simulink model "five_bar_model_v_1"  (R2018a)
settings: Solver=ode45  StartTime=0.0  StopTime=tmax  FixedStep=0.0001  MaxStep=1e-4  RelTol=1e-3
values from neighbouring files (symbols this model uses):
  dt = 10e-3    (= 0.01)    [model_parameters_v_1.m]    (also in test_dynamics.m = 0.2; test_kinematics.m = 0.1)
  g = -9.80665    [idyn5.m]    (also in test_dynamics.m; test_model.m = 9.80665)
  Kd = (3*aj*wj-Fv) * eye(2)    [model_parameters_v_1.m]
  Kdi = [2 * zita *  wpos1; 2  * zita * wpos2]    [model_parameters_v_1.m]
  Ki = aj*wj^3 * eye(2)    [model_parameters_v_1.m]
  Kp = 3*aj*wj^2 * eye(2)    [model_parameters_v_1.m]
  Kpi = [ wpos1^2;  wpos2^2]    [model_parameters_v_1.m]
  p = [NaN; NaN]    [fkine5.m]    (also in test_model.m = zeros(n,2))
  q = [NaN; NaN; NaN; NaN; NaN]    [fkine5.m]    (also in ikine5.m = [q11;q12;q13;q21;q22])
  q0 = q(:,1)    [model_parameters_v_1.m]    (also in test_dynamics.m = q0(:,4); test_kinematics.m = q0(:,4))
  qd = [qda(1);qdu(1);qdu(2);qda(2);qdu(3)]    [ifirstkine5.m]
  qdd = [qdda(1);qddu(1);qddu(2);qdda(2);qddu(3)]    [isecondkine5.m]
  t0r = J * qda    [ffirstkine5.m]    (also in test_dynamics.m = [0;0]; test_kinematics.m = [1;1]; test_model.m = p)
  t0rd = (J * qdda+ at)    [fsecondkine5.m]    (also in test_dynamics.m = [0;0]; test_kinematics.m = [-1;1]; test_model.m = p)
undefined symbols (not defined in the file or in its folder): Kii, tmax, X, Y, Z
libraries: sm_lib x24, simulink x12, nesl_utility x9, powerlib_meascontrol x2
(part 2 of 2)

== matlab function five_bar_model_v_1/five-bar-robot1/direct dynamic ==
  data: T input; qdda output; q input; qd input; J input; Jt input; Jta input; Jtd input; Psit input; atp input; ad input; Tl input
function qdda  = ddyn5(T,q,qd,J,Jt,Jta,Jtd,Psit,atp,ad, Tl)
    l = 0.205;
    d1 = [-0.125, l, l];
    d2 = [0.125, l, l];
    q1 = q(1:3);
    q2 = q(4:5);
    qd1 = qd(1:3);
    qd2 = qd(4:5);
    % Numerical Solution Dynamics
    % Gravity 
%     g = -9.80665;
    g = 0;
    
   % Dynamics parameters
    m11 = 0.126; %kg
    mx11 = m11 * 0.1025;
    my11 =  0; %m11 * 1.44e-2;
    zz11 = 0.001774; %kg-m^2;
    
    m12 = 0.126; %kg
    mx12 = m12 * 0.1025;
    my12 =  0; %m11 * 1.44e-2;
    zz12 = 0.001774; %kg-m^2;
    
    m21 = 0.126; %kg
    mx21 = m21 * 0.1025;
    my21 =  0; %m11 * 1.44e-2;
    zz21 = 0.001774; %kg-m^2;
    
    m22 = 0.126; %kg
    mx22 = m22 * 0.1025;
    my22 =  0; %m11 * 1.44e-2;
    zz22 = 0.001774; %kg-m^2;
    
    Ia11 = 4.8e-5; % kg-m2
    zz11r = zz11 + Ia11 + d1(2)^2 * m12;
    
    Ia21 = 4.8e-5; % kg-m2
    zz21r = zz21 + Ia21 + d2(2)^2 * m22;
   
    %Fricciones fv = viscosa fs= seca
    fv1 = [1.5e-1 0 0];
    fs1 = [1.5e-1 0 0];
    fv2 = [0 0];
    fs2 = [0 0];
    % End effector mass
    m4 = 0.272;
    
    % Direct dynamics model
    M11 = zz11r + zz12 + 2 * d1(2) * mx12 * cos(q1(2)) - ...
          2 * d1(2) * my12 * sin(q1(2));

    M12 = zz12 + d1(2) * mx12 * cos(q1(2)) - ...
          d1(2) * my12 * sin(q1(2));
    M21 = M12;

    M44 = zz21r + zz22 + 2 * d2(2) * mx22 * cos(q2(2)) - ...
          2 * d2(2) * my22 * sin(q2(2));

    M45 = zz22 + d2(2) * mx22 * cos(q2(2)) - ...
          d2(2) * my22 * sin(q2(2));
    M54 = M45;

    Mt = [M11 M12  0 0     0;
          M21 zz12 0 0     0;
          0   0    0 0     0;
          0   0    0 M44 M45;
          0   0    0 M54 zz22];

    c1 = -d1(2) * mx12 * qd1(2) * (2 * qd1(1) + qd1(2)) * sin(q1(2)) ...
         -d1(2) * my12 * qd1(2) * (2 * qd1(1) + qd1(2)) * cos(q1(2)) ...
         +fs1(1) * sign(qd1(1)) + fv1(1) * qd1(1) ...
         +(my12*sin(q1(1) + q1(2)) - mx12*cos(q1(1) + q1(2)) ...
         - mx11*cos(q1(1)) + my11*sin(q1(1)) - d1(2)*m12*cos(q1(1)))*g;

    c2 = d1(2) * mx12 * qd1(1)^2 * sin(q1(2)) ...
         +d1(2) * my12 * qd1(1)^2 * cos(q1(2)) ...
         +fs1(2) * sign(qd1(2)) + fv1(2) * qd1(2) ...
         +(my12*sin(q1(1) + q1(2)) - mx12*cos(q1(1) + q1(2)))*g;

    c3 = fs1(3)*sign(qd1(3)) + fv1(3)*qd1(3);

    c4 = -d2(2) * mx22 * qd2(2) * (2 * qd2(1) + qd2(2)) * sin(q2(2)) ...
         -d2(2) * my22 * qd2(2) * (2 * qd2(1) + qd2(2)) * cos(q2(2)) ...
         +fs2(1) * sign( qd2(1) ) + fv2(1) * qd2(1) ...
         +(my22*sin(q2(1) + q2(2)) - mx22*cos(q2(1) + q2(2)) ...
         -mx21*cos(q2(1)) + my21*sin(q2(1)) - d2(2)*m22*cos(q2(1)))*g;

    c5 = d2(2) * mx22 * qd2(1)^2 * sin(q2(2)) ...
         +d2(2) * my22 * qd2(1)^2 * cos(q2(2)) ...
         +fs2(2) * sign(qd2(2)) + fv2(2) * qd2(2) ...
         +(my22*sin(q2(1) + q2(2)) - mx22*cos(q2(1) + q2(2)))*g;

    ct = [c1; c2; c3; c4; c5];

    Et = [1 0 0 0 0;
          0 0 1 0 0;
          0 0 0 1 0;
          0 1 0 0 0;
          0 0 0 0 1];

    M0p = m4 * [eye(2), zeros(2,4); zeros(4,2), zeros(4)];
    % c0p = zeros(6,1); 
    c0p = m4*[0;-g;0;0;0;0]; 
%     J'*Psit'*(c0p)
    % M0r = Psit' * M0p * Psit; % Igual a m4*eye(2)
    M0r = m4 * eye(2);

    Jd = Jtd \ (Jt * J - Jta);

    M = [eye(2), Jd'] * Et'*Mt*Et * [eye(2);Jd] + J'*M0r*J;

    c0r = M0p * atp; % Debe ser igual a 0

    c = [eye(2) Jd'] * Et' * (ct + Mt*Et*[zeros(2,1); ad]) ...
        + J'*Psit'*(c0r+c0p); % if c0r and c0p are 0 the second term is 0

    qdda = pinv(M) * (T-c-Tl);

== matlab function five_bar_model_v_1/five-bar-robot1/passive velocities ==
  data: qda input; p input; q input; qd output; qdp output; t0r output; Ar output; J output; Jinv output; Jt output; Jta output; Jtd output; Psit output
function [qd,qdp,t0r,Ar,J,Jinv,Jt,Jta,Jtd,Psit] = passive_velocities5(qda,p,q)
%% This function compute the passive velocities of the joints
% @param t0r: twist end-effector vector 2X1
% @param p: end-effector coordinate vector 2X1
% @param q: joint positions vector 5x1
% @return qd: velocity joints vector 5x1
% @return qda: active velocity joints vector 2X1
% @return qdu: underactuated velocity joints vector 3X1
% @return Ar: matrix 2x2 relates the n dof independent coordinates of the platform twist 0 t r to the actuated joints q̇ a
% @return B: matrix 2x2 for computation of the dynamic model of the PKM
% @return J: kinematic Jacobian matrix of the PKM
% @return Jinv: inverse kinematic Jacobian matrix of the PKM
% @return Jt: crucial for computation of the dynamic model of the PKM.
% @return Jta: crucial for computation of the dynamic model of the PKM.
% @return Jtd: crucial for computation of the dynamic model of the PKM.
% @return Psit: matrix 2X6
%%
    l = 0.205;
    d1 = [-0.125, l, l];
    d2 = [0.125, l, l];
    q1 = q(1:3);
    q2 = q(4:5);
    Phi = sum(q1);
    x = p(1);
    y = p(2);

    B = -[ d1(2)*sin(q1(2)), 0;
          0, d2(2)*sin(q2(2))];


    Ar = [cos(q1(1) + q1(2)), sin(q1(1) + q1(2));
          cos(q2(1) + q2(2)), sin(q2(1) + q2(2))];
    % forward model
    J = -pinv(Ar) * B;
    t0r = J * qda;
    % t0r =[ -(d1(2)*qd11*sin(q2(1) + q2(2))*sin(q1(2)) - ...
    %                 d2(2)*qd21*sin(q1(1) + q1(2))*sin(q2(2)))/sin(q1(1) + q1(2) - q2(1) - q2(2));
    %         (d1(2)*qd11*cos(q2(1) + q2(2))*sin(q1(2)) - ...
    %                 d2(2)*qd21*cos(q1(1) + q1(2))*sin(q2(2)))/sin(q1(1) + q1(2) - q2(1) - q2(2))];

    Jinv = -pinv(B) * Ar;
%     qda = Jinv * t0r;
    % qda = [(xd*cos(q1(1) + q1(2)) + yd*sin(q1(1) + q1(2)))/(d1(2)*sin(q1(2)));
    %        (xd*cos(q2(1) + q2(2)) + yd*sin(q2(1) + q2(2)))/(d2(2)*sin(q2(2)))];

    % passive velocities calculation

    ay = cos(Phi)^2 / (x - d2(2)*cos(q2(1)) - d2(1));
    ax = - ((y-d2(2)*sin(q2(1)))*cos(Phi)^2) ...
           / (x - d2(2)*cos(q2(1)) - d2(1))^2;
    aq = -(d2(2) * ((x-d2(1))*cos(q2(1)) ...
          +y*sin(q2(1))-d2(2))*cos(Phi)^2) ...
          / (x - d2(2)*cos(q2(1)) - d2(1))^2;

    Psit = [1                     0
            0                     1
            0                     0
            0                     0
            0                     0
            (ax+aq*Jinv(2,1)) (ay+aq*Jinv(2,2))];

    Jt = [-sin(q1(1) + q1(2)),cos(q1(1) + q1(2));
            (ax + aq*Jinv(2,1)), (ay + aq*Jinv(2,2));
            -sin(q2(1) + q2(2)),cos(q2(1) + q2(2))];


    Jta = [ d1(3) + d1(2)*cos(q1(2)), 0;
            1,                0;
            0,      d2(3) + d2(2)*cos(q2(2))];

    Jtd = [ d1(3), 0,   0;
            1,   1,   0;
            0,   0, d2(3)];

    qdp = Jtd\(Jt * t0r - Jta * qda);
    qd = [qda(1);qdp(1);qdp(2);qda(2);qdp(3)];

== matlab function five_bar_model_v_1/five-bar-robot1/second order inverse kinematics ==
  data: qdda input; qdd output; t0r input; p input; q input; qd input; Ar input; J input; Jinv input; Jt input; Jta input; Jtd input; Psit input; qddp output; t0rd output; Psit1 output; Psit2 output; atp output; ad output
function [qdd,qddp,t0rd,Psit1,Psit2,atp,ad] = passive_acc5(qdda,t0r,p,q,qd,Ar,J,Jinv,Jt,Jta,Jtd,Psit)
% This function implement the second-order inverse kinematics model of a five bar robot
% @param t0rd: derivate twist end-effector vector 2X1
% @param t0r: twist end-effector vector 2X1
% @param p: end-effector coordinate vector 2X1
% @param q: joint positions vector 5x1
% @param qd: velocity joints vector 5x1
% @param Ar: matrix 2x2 for computation of the dynamic model of the PKM
% @param B: matrix 2x2 for computation of the dynamic model of the PKM
% @param Jinv: inverse kinematic Jacobian matrix of the PKM
% @param Jt: crucial for computation of the dynamic model of the PKM.
% @param Jta: crucial for computation of the dynamic model of the PKM.
% @param Jtd: crucial for computation of the dynamic model of the PKM.
% @return qdd: acceleration joint vector 5x1
% @return qdda: active acceleration joints vector 2X1
% @return qddu: underactuated acceleration joints vector 3X1
% @return Psit1: matrix 2x6
% @return Psit2: matrix 1x6
% @return atp: acceleration using for dynamics
% @return ad: acceleration using for dynamics

    l = 0.205;
    d1 = [-0.125, l, l];
    d2 = [0.125, l, l];
    q1 = q(1:3);
    q2 = q(4:5);
    qd1 = qd(1:3);
    qd2 = qd(4:5);
    Phi = sum(q1);
    Phid = sum(qd1);
    x = p(1);
    y = p(2);
    xd = t0r(1);
    yd = t0r(2);

    wr1 = [cos(q1(1)+q1(2)); sin(q1(1)+q1(2)); 0; 0; 0; 0];
    wr2 = [cos(q2(1)+q2(2)); sin(q2(1)+q2(2)); 0; 0; 0; 0];

    b01a_ = [-d1(2)*qd1(1)*cos(q1(1)) - d1(3)*cos(q1(1)+q1(2))*(qd1(1)+qd1(2));
             -d1(2)*qd1(1)*sin(q1(1)) - d1(3)*sin(q1(1)+q1(2))*(qd1(1)+qd1(2));
             zeros(4,1)];
    b01b_ = [-d1(3)*cos(q1(1)+q1(2));
             -d1(3)*sin(q1(1)+q1(2));
             zeros(4,1)];
    b0p1 = b01a_ * qd1(1) + b01b_ * qd1(2)*(qd1(1)+qd1(2));

    b02a_ = [-d2(2)*qd2(1)*cos(q2(1)) - d2(3)*cos(q2(1)+q2(2))*(qd2(1)+qd2(2));
             -d2(2)*qd2(1)*sin(q2(1)) - d2(3)*sin(q2(1)+q2(2))*(qd2(1)+qd2(2));
             zeros(4,1)];
    b02b_ = [-d2(3)*cos(q2(1)+q2(2));
             -d2(3)*sin(q2(1)+q2(2));
             zeros(4,1)];
    b0p2 = b02a_ * qd2(1) + b02b_ * qd2(2)*(qd2(1)+qd2(2));

    b0p = [(wr1'*b0p1); (wr2'*b0p2)];

%     aqq = pinv(B) * b0p;
    at = pinv(Ar) * b0p;
    t0rd = (J * qdda + at);
%     qdda = (Jinv * t0rd + aqq);

    % Aceleracion pasiva

    ayd = (Phid*sin(2*Phi))/(d2(1) - x + d2(2)*cos(q2(1))) - (cos(Phi)^2*(xd + d2(2)*qd2(1)*sin(q2(1))))/(d2(1) - x + d2(2)*cos(q2(1)))^2;

    axd = (Phid*sin(2*Phi)*(y - d2(2)*sin(q2(1))))/(d2(1) - x + d2(2)*cos(q2(1)))^2 ...
        - (cos(Phi)^2*(yd - d2(2)*qd2(1)*cos(q2(1))))/(d2(1) - x + d2(2)*cos(q2(1)))^2 ...
        - (2*cos(Phi)^2*(xd + d2(2)*qd2(1)*sin(q2(1)))*(y - d2(2)*sin(q2(1))))/(d2(1) - x + d2(2)*cos(q2(1)))^3;

    aqd = (2*d2(2)*cos(Phi)^2*(xd + d2(2)*qd2(1)*sin(q2(1)))*(d2(2) - sin(q2(1))*y + cos(q2(1))*(d2(1) - x)))...
        /(d2(1) - x + d2(2)*cos(q2(1)))^3 ...
        - (d2(2)*cos(Phi)^2*(xd*cos(q2(1)) + yd*sin(q2(1)) + qd2(1)*cos(q2(1))*y + qd2(1)*sin(q2(1))*(d2(1) - x)))...
        /(d2(1) - x + d2(2)*cos(q2(1)))^2 ...
        - (2*Phid*d2(2)*cos(Phi)*sin(Phi)*(d2(2) - sin(q2(1))*y + cos(q2(1))*(d2(1) - x)))...
        /(d2(1) - x + d2(2)*cos(q2(1)))^2;

    j21_invd = -(sin(q2(1) + q2(2))*(qd2(1) + qd2(2)))/(d2(2)*sin(q2(2))) ...
               -(qd2(2)*cos(q2(1) + q2(2))*cos(q2(2)))/(d2(2)*sin(q2(2))^2);

    j22_invd = -(qd2(2)*sin(q2(1) + q2(2))*cos(q2(2)))/(d2(2)*sin(q2(2))^2) ...
               +(cos(q2(1) + q2(2))*(qd2(1) + qd2(2)))/(d2(2)*sin(q2(2)));

    aq = -(d2(2) * ((x-d2(1))*cos(q2(1))+y*sin(q2(1))-d2(2))*cos(Phi)^2) / (x - d2(2)*cos(q2(1)) - d2(1))^2;

    psitd1 = axd + aqd*Jinv(2,1)+ aq*j21_invd;
    psitd2 = ayd + aqd*Jinv(2,2)+ aq*j22_invd;

    Psidt = [0 0; 0 0; 0 0; 0 0; 0 0; psitd1 psitd2];

    Psit1 = [-sin(q1(1)+q1(2)) cos(q1(1)+q1(2)) 0 0 0 0
             0                 0                0 0 0 1];
    Psit2 = [-sin(q2(1)+q2(2)) cos(q2(1)+q2(2)) 0 0 0 0];

    dc1 = Psit1 * (eye(6)* Psidt * t0r - b0p1); % Jti = I6x6 -> di = 06x1
    dc2 = Psit2 * (eye(6)* Psidt * t0r - b0p2);
    dc = [dc1; dc2];

    qddp =  Jtd\(Jt*t0rd - Jta*qdda + dc);

    qdd = [qdda(1);qddp(1);qddp(2);qdda(2);qddp(3)];

    at = pinv(Ar) * b0p;
    atp = Psit * at + Psidt * t0r;% using for dynamics
    ad = Jtd \ (dc + Jt*at); % For dynamics

== matlab function five_bar_model_v_1/five-bar-robot1/forward kinematics ==
  data: qa input; p output; assembly input; q output
function [p,q] = fkine5(qa, assembly)
% This function implement the forward kinematic model of a five bar robot
% @parm qa: active joint positions vector 2x1
% @parm assembly: assembly mode selecction 1 for + -1 for -
% @return p: p end-effector coordinate vector 2X1
% @return q: joint positon vector 5X1
    l = 0.205;
    d1 = [-0.125, l, l];
    d2 = [0.125, l, l];
    q11 = qa(1);
    q21 = qa(2);

    A12 = [d1(2)*cos(q11)+d1(1); d1(2)*sin(q11)];
    A22 = [d2(2)*cos(q21)+d2(1); d2(2)*sin(q21)];

    if sqrt((A12-A22)' * (A12-A22)) <= 2*l
        a1 = - 2*d1(1) - 2*d1(2)*cos(q11);
        a2 = - 2*d2(1) - 2*d2(2)*cos(q21);
        b1 = - 2*sin(q11)*d1(2);
        b2 = - 2*sin(q21)*d2(2);
        c1 = d1(1)^2 + 2*cos(q11)*d1(1)*d1(2) + d1(2)^2 - d1(3)^2;
        c2 = d2(1)^2 + 2*cos(q21)*d2(1)*d2(2) + d2(2)^2 - d2(3)^2;

        if b1 ~= b2
            a = a2 - a1;
            b = b2 - b1;
            c = c2 - c1;
            e1 = - a / b;
            e2 = - c / b;
            f1 = 1 + e1^2;
            f2 = 2 * e1 * e2 + a1 + b1 * e1;
            f3 = e2^2 + b1 * e2 + c1;

            x = (-f2 - sqrt(f2^2 - 4 * f1 * f3)) / (2 * f1);
            y = e1 * x + e2;

            A13=[x-A12(1);y-A12(2)];
            A23=[x-A22(1);y-A22(2)];
            if  A13(1)*A23(2)-A23(1)*A13(2) <= 0 && assembly == 1
                x = (-f2 + sqrt(f2^2 - 4 * f1 * f3)) / (2 * f1);
                y = e1 * x + e2;
            elseif  A13(1)*A23(2)-A23(1)*A13(2) >= 0 && assembly == -1
                x = (-f2 + sqrt(f2^2 - 4 * f1 * f3)) / (2 * f1);
                y = e1 * x + e2;
            end
        else
            x = - (c2 - c1) / (a2 - a1);
            y = (-b1 + (b1^2 - 4 * (x^2 + a1 * x + c1))^(1/2)) / 2;

            A13=[x-A12(1);y-A12(2)];
            A23=[x-A22(1);y-A22(2)];
            if  A13(1)*A23(2)-A23(1)*A13(2) <= 0 && assembly == 1
                y = (-b1 - (b1^2 - 4 * (x^2 + a1 * x + c1))^(1/2)) / 2;
            elseif  A13(1)*A23(2)-A23(1)*A13(2) >= 0 && assembly == -1
                y = (-b1 - (b1^2 - 4 * (x^2 + a1 * x + c1))^(1/2)) / 2;
            end
        end

        % for q12 and q22 from a12/a11 and a22/a21
        q12 = atan2(y-d1(2)*sin(q11), x-d1(1)-d1(2)*cos(q11)) - q11;
        q22 = atan2(y-d2(2)*sin(q21), x-d2(1)-d2(2)*cos(q21)) - q21;
        q13 = q21 + q22 - q11 - q12;
        p = [x;y];
        q = [q11; q12; q13; q21; q22];
        
        % I will work in the first assembly.
        % Note: A way of implement the change of assembly is using the equations
        % (3) and (4) of the paper Minimum-time trajectory planning and control
        % of a pick-and-place five-bar parallel robot. Obtaining the
        % previous assembly, then the current and finally comparing
        % eache other.
%         sum(angdiff(q, q_prev).^2)
%         if sum(angdiff(q, q_prev).^2) > 0.1 
%             disp('Atention!!');
%             assembly2 = -assembly;
%             q11 = qa(1);
%             q21 = qa(2);
%             a1 = - 2*d1(1) - 2*d1(2)*cos(q11);
%             a2 = - 2*d2(1) - 2*d2(2)*cos(q21);
%             b1 = - 2*sin(q11)*d1(2);
%             b2 = - 2*sin(q21)*d2(2);
%             c1 = d1(1)^2 + 2*cos(q11)*d1(1)*d1(2) + d1(2)^2 - d1(3)^2;
%             c2 = d2(1)^2 + 2*cos(q21)*d2(1)*d2(2) + d2(2)^2 - d2(3)^2;
% 
%             if b1 ~= b2
%                 a = a2 - a1;
%                 b = b2 - b1;
%                 c = c2 - c1;
%                 e1 = - a / b;
%                 e2 = - c / b;
%                 f1 = 1 + e1^2;
%                 f2 = 2 * e1 * e2 + a1 + b1 * e1;
%                 f3 = e2^2 + b1 * e2 + c1;
% 
%                 x = (-f2 - sqrt(f2^2 - 4 * f1 * f3)) / (2 * f1);
%                 y = e1 * x + e2;
% 
%                 A13=[x-A12(1);y-A12(2)];
%                 A23=[x-A22(1);y-A22(2)];
%                 if  A13(1)*A23(2)-A23(1)*A13(2) <= 0 && assembly2 == 1
%                     x = (-f2 + sqrt(f2^2 - 4 * f1 * f3)) / (2 * f1);
%                     y = e1 * x + e2;
%                 elseif  A13(1)*A23(2)-A23(1)*A13(2) >= 0 && assembly2 == -1
%                     x = (-f2 + sqrt(f2^2 - 4 * f1 * f3)) / (2 * f1);
%                     y = e1 * x + e2;
%                 end
%             else
%                 x = - (c2 - c1) / (a2 - a1);
%                 y = (-b1 + (b1^2 - 4 * (x^2 + a1 * x + c1))^(1/2)) / 2;
% 
%                 A13=[x-A12(1);y-A12(2)];
%                 A23=[x-A22(1);y-A22(2)];
%                 if  A13(1)*A23(2)-A23(1)*A13(2) <= 0 && assembly == 1
%                     y = (-b1 - (b1^2 - 4 * (x^2 + a1 * x + c1))^(1/2)) / 2;
%                 elseif  A13(1)*A23(2)-A23(1)*A13(2) >= 0 && assembly == -1
%                     y = (-b1 - (b1^2 - 4 * (x^2 + a1 * x + c1))^(1/2)) / 2;
%                 end
%             end
% 
%             % for q12 and q22 from a12/a11 and a22/a21
%             q12 = atan2(y-d1(2)*sin(q11), x-d1(1)-d1(2)*cos(q11)) - q11;
%             q22 = atan2(y-d2(2)*sin(q21), x-d2(1)-d2(2)*cos(q21)) - q21;
%             q13 = q21 + q22 - q11 - q12;
%             p = [x;y];
%             q = [q11; q12; q13; q21; q22];
%         end
    else
        disp('ERROR: Euclidian distance > 2*l');
        p = [NaN; NaN];
        q = [NaN; NaN; NaN; NaN; NaN];
    end

== matlab function five_bar_model_v_1/Inverse dynamic control/inverse dynamics ==
  data: q input; T output double size=2; qd input; qdda input; qddp input; t0rd input; J input; Jt input; Jta input; Jtd input; Psit input
function T  = idyn5(q,qd,qdda,qddp,t0rd,J,Jt,Jta,Jtd,Psit)

    l = 0.205;
    d1 = [-0.125, l, l];
    d2 = [0.125, l, l];
    q1 = q(1:3);
    q2 = q(4:5);
    qd1 = qd(1:3);
    qd2 = qd(4:5);
    qdd1 = [qdda(1);qddp(1:2)];
    qdd2 = [qdda(2);qddp(3)];
    xdd = t0rd(1);
    ydd = t0rd(2);
    Tt1 = zeros(3,1);
    Tt2 = zeros(2,1);
    Ttd = zeros(3,1);
    % Dynamic
    % Gravity 
%     g = -9.80665;
    g = 0;
% Dynamics parameters
    m11 = 0.126; %kg
    mx11 = m11 * 0.1025;
    my11 =  0; %m11 * 1.44e-2;
    zz11 = 0.001774; %kg-m^2;
    
    m12 = 0.126; %kg
    mx12 = m12 * 0.1025;
    my12 =  0; %m11 * 1.44e-2;
    zz12 = 0.001774; %kg-m^2;
    
    m21 = 0.126; %kg
    mx21 = m21 * 0.1025;
    my21 =  0; %m11 * 1.44e-2;
    zz21 = 0.001774; %kg-m^2;
    
    m22 = 0.126; %kg
    mx22 = m22 * 0.1025;
    my22 =  0; %m11 * 1.44e-2;
    zz22 = 0.001774; %kg-m^2;
    
    Ia11 = 4.8e-5; % kg-m2
%     zz11r = zz11 + Ia11 + d1(2)^2 * m12;
    
    Ia21 = 4.8e-5; % kg-m2
%     zz21r = zz21 + Ia21 + d2(2)^2 * m22;
   
    %Fricciones fv = viscosa fs= seca
    fv1 = [1.5e-1 0 0];
    fs1 = [1.5e-1 0 0];
    fv2 = [0 0];
    fs2 = [0 0];
    % End effector mass
    m4 = 0.272;

    % Inverse dynamics model
    Tt1(1) = (my12*sin(q1(1) + q1(2)) - mx12*cos(q1(1) + q1(2)) ...
        - mx11*cos(q1(1)) + my11*sin(q1(1)) - d1(2)*m12*cos(q1(1)))*g ...
        + Ia11*qdd1(1) + fv1(1)*qd1(1) + fs1(1)*sign(qd1(1)) ...
        + mx12*(- d1(2)*sin(q1(2))*qd1(2)^2 - 2*d1(2)*qd1(1)*sin(q1(2))*qd1(2) ...
        + 2*d1(2)*qdd1(1)*cos(q1(2)) + d1(2)*qdd1(2)*cos(q1(2))) ...
        - my12*(d1(2)*cos(q1(2))*qd1(2)^2 + 2*d1(2)*qd1(1)*cos(q1(2))*qd1(2) ...
        + 2*d1(2)*qdd1(1)*sin(q1(2)) + d1(2)*qdd1(2)*sin(q1(2))) ...
        + qdd1(1)*zz11 + qdd1(1)*zz12 + qdd1(2)*zz12 + m12*qdd1(1)*d1(2)^2;
    Tt1(2) = (my12*sin(q1(1) + q1(2)) - mx12*cos(q1(1) + q1(2)))*g ...
        + zz12*(qdd1(1) + qdd1(2)) + fv1(2)*qd1(2) + fs1(2)*sign(qd1(2)) ...
        + mx12*(d1(2)*sin(q1(2))*qd1(1)^2 + d1(2)*qdd1(1)*cos(q1(2))) ...
        - my12*(-d1(2)*cos(q1(2))*qd1(1)^2 + d1(2)*qdd1(1)*sin(q1(2)));
    Tt1(3) = fs1(3) * sign(qd1(3)) + fv1(3)*qd1(3);
    
    Tt2(1) = (my22*sin(q2(1) + q2(2)) - mx22*cos(q2(1) + q2(2)) ...
        - mx21*cos(q2(1)) + my21*sin(q2(1)) - d2(2)*m22*cos(q2(1)))*g ...
        + Ia21*qdd2(1) + fv2(1)*qd2(1) + fs2(1)*sign(qd2(1)) ...
        + mx22*(- d2(2)*sin(q2(2))*qd2(2)^2 - 2*d2(2)*qd2(1)*sin(q2(2))*qd2(2) ...
        + 2*d2(2)*qdd2(1)*cos(q2(2)) + d2(2)*qdd2(2)*cos(q2(2))) ...
        - my22*(d2(2)*cos(q2(2))*qd2(2)^2 + 2*d2(2)*qd2(1)*cos(q2(2))*qd2(2) ...
        + 2*d2(2)*qdd2(1)*sin(q2(2)) + d2(2)*qdd2(2)*sin(q2(2))) ...
        + qdd2(1)*zz21 + qdd2(1)*zz22 + qdd2(2)*zz22 + m22*qdd2(1)*d2(2)^2;
   
    Tt2(2) = (my22*sin(q2(1) + q2(2)) - mx22*cos(q2(1) + q2(2)))*g ...
        + zz22*(qdd2(1) + qdd2(2)) + fv2(2)*qd2(2) + fs2(2)*sign(qd2(2)) ...
        + mx22*(d2(2)*sin(q2(2))*qd2(1)^2 + d2(2)*qdd2(1)*cos(q2(2))) ...
        - my22*(-d2(2)*cos(q2(2))*qd2(1)^2 + d2(2)*qdd2(1)*sin(q2(2)));

    % End effector like a punctual mass fixed on B22
    w0p = m4 * [xdd; ydd-g; zeros(4,1)];
    w0r = Psit' * w0p;
    % IDM
    Tta = [Tt1(1); Tt2(1)];
    Ttd = [Tt1(2:3); Tt2(2)];

    Jd = (Jtd) \ (Jt * J - Jta);

    T = Tta + J' * w0r + Jd' * Ttd;

== matlab function five_bar_model_v_1/five-bar-robot2/direct dynamic ==
  data: T input; qdda output; q input; qd input; J input; Jt input; Jta input; Jtd input; Psit input; atp input; ad input; Tl input
function qdda  = ddyn5(T,q,qd,J,Jt,Jta,Jtd,Psit,atp,ad, Tl)
    l = 0.205;
    d1 = [-0.125, l, l];
    d2 = [0.125, l, l];
    q1 = q(1:3);
    q2 = q(4:5);
    qd1 = qd(1:3);
    qd2 = qd(4:5);
    % Numerical Solution Dynamics
    % Gravity 
%     g = -9.80665;
    g = 0;
    
   % Dynamics parameters
    m11 = 0.126; %kg
    mx11 = m11 * 0.1025;
    my11 =  0; %m11 * 1.44e-2;
    zz11 = 0.001774; %kg-m^2;
    
    m12 = 0.126; %kg
    mx12 = m12 * 0.1025;
    my12 =  0; %m11 * 1.44e-2;
    zz12 = 0.001774; %kg-m^2;
    
    m21 = 0.126; %kg
    mx21 = m21 * 0.1025;
    my21 =  0; %m11 * 1.44e-2;
    zz21 = 0.001774; %kg-m^2;
    
    m22 = 0.126; %kg
    mx22 = m22 * 0.1025;
    my22 =  0; %m11 * 1.44e-2;
    zz22 = 0.001774; %kg-m^2;
    
    Ia11 = 4.8e-5; % kg-m2
    zz11r = zz11 + Ia11 + d1(2)^2 * m12;
    
    Ia21 = 4.8e-5; % kg-m2
    zz21r = zz21 + Ia21 + d2(2)^2 * m22;
   
    %Fricciones fv = viscosa fs= seca
    fv1 = [1.5e-1 0 0];
    fs1 = [1.5e-1 0 0];
    fv2 = [0 0];
    fs2 = [0 0];
    % End effector mass
    m4 = 0.272;
    
    % Direct dynamics model
    M11 = zz11r + zz12 + 2 * d1(2) * mx12 * cos(q1(2)) - ...
          2 * d1(2) * my12 * sin(q1(2));

    M12 = zz12 + d1(2) * mx12 * cos(q1(2)) - ...
          d1(2) * my12 * sin(q1(2));
    M21 = M12;

    M44 = zz21r + zz22 + 2 * d2(2) * mx22 * cos(q2(2)) - ...
          2 * d2(2) * my22 * sin(q2(2));

    M45 = zz22 + d2(2) * mx22 * cos(q2(2)) - ...
          d2(2) * my22 * sin(q2(2));
    M54 = M45;

    Mt = [M11 M12  0 0     0;
          M21 zz12 0 0     0;
          0   0    0 0     0;
          0   0    0 M44 M45;
          0   0    0 M54 zz22];

    c1 = -d1(2) * mx12 * qd1(2) * (2 * qd1(1) + qd1(2)) * sin(q1(2)) ...
         -d1(2) * my12 * qd1(2) * (2 * qd1(1) + qd1(2)) * cos(q1(2)) ...
         +fs1(1) * sign(qd1(1)) + fv1(1) * qd1(1) ...
         +(my12*sin(q1(1) + q1(2)) - mx12*cos(q1(1) + q1(2)) ...
         - mx11*cos(q1(1)) + my11*sin(q1(1)) - d1(2)*m12*cos(q1(1)))*g;

    c2 = d1(2) * mx12 * qd1(1)^2 * sin(q1(2)) ...
         +d1(2) * my12 * qd1(1)^2 * cos(q1(2)) ...
         +fs1(2) * sign(qd1(2)) + fv1(2) * qd1(2) ...
         +(my12*sin(q1(1) + q1(2)) - mx12*cos(q1(1) + q1(2)))*g;

    c3 = fs1(3)*sign(qd1(3)) + fv1(3)*qd1(3);

    c4 = -d2(2) * mx22 * qd2(2) * (2 * qd2(1) + qd2(2)) * sin(q2(2)) ...
         -d2(2) * my22 * qd2(2) * (2 * qd2(1) + qd2(2)) * cos(q2(2)) ...
         +fs2(1) * sign( qd2(1) ) + fv2(1) * qd2(1) ...
         +(my22*sin(q2(1) + q2(2)) - mx22*cos(q2(1) + q2(2)) ...
         -mx21*cos(q2(1)) + my21*sin(q2(1)) - d2(2)*m22*cos(q2(1)))*g;

    c5 = d2(2) * mx22 * qd2(1)^2 * sin(q2(2)) ...
         +d2(2) * my22 * qd2(1)^2 * cos(q2(2)) ...
         +fs2(2) * sign(qd2(2)) + fv2(2) * qd2(2) ...
         +(my22*sin(q2(1) + q2(2)) - mx22*cos(q2(1) + q2(2)))*g;

    ct = [c1; c2; c3; c4; c5];

    Et = [1 0 0 0 0;
          0 0 1 0 0;
          0 0 0 1 0;
          0 1 0 0 0;
          0 0 0 0 1];

    M0p = m4 * [eye(2), zeros(2,4); zeros(4,2), zeros(4)];
    % c0p = zeros(6,1); 
    c0p = m4*[0;-g;0;0;0;0]; 
%     J'*Psit'*(c0p)
    % M0r = Psit' * M0p * Psit; % Igual a m4*eye(2)
    M0r = m4 * eye(2);

    Jd = Jtd \ (Jt * J - Jta);

    M = [eye(2), Jd'] * Et'*Mt*Et * [eye(2);Jd] + J'*M0r*J;

    c0r = M0p * atp; % Debe ser igual a 0

    c = [eye(2) Jd'] * Et' * (ct + Mt*Et*[zeros(2,1); ad]) ...
        + J'*Psit'*(c0r+c0p); % if c0r and c0p are 0 the second term is 0

    qdda = pinv(M) * (T-c-Tl);

== matlab function five_bar_model_v_1/five-bar-robot2/passive velocities ==
  data: qda input; p input; q input; qd output; qdp output; t0r output; Ar output; J output; Jinv output; Jt output; Jta output; Jtd output; Psit output
function [qd,qdp,t0r,Ar,J,Jinv,Jt,Jta,Jtd,Psit] = passive_velocities5(qda,p,q)
%% This function compute the passive velocities of the joints
% @param t0r: twist end-effector vector 2X1
% @param p: end-effector coordinate vector 2X1
% @param q: joint positions vector 5x1
% @return qd: velocity joints vector 5x1
% @return qda: active velocity joints vector 2X1
% @return qdu: underactuated velocity joints vector 3X1
% @return Ar: matrix 2x2 relates the n dof independent coordinates of the platform twist 0 t r to the actuated joints q̇ a
% @return B: matrix 2x2 for computation of the dynamic model of the PKM
% @return J: kinematic Jacobian matrix of the PKM
% @return Jinv: inverse kinematic Jacobian matrix of the PKM
% @return Jt: crucial for computation of the dynamic model of the PKM.
% @return Jta: crucial for computation of the dynamic model of the PKM.
% @return Jtd: crucial for computation of the dynamic model of the PKM.
% @return Psit: matrix 2X6
%%
    l = 0.205;
    d1 = [-0.125, l, l];
    d2 = [0.125, l, l];
    q1 = q(1:3);
    q2 = q(4:5);
    Phi = sum(q1);
    x = p(1);
    y = p(2);

    B = -[ d1(2)*sin(q1(2)), 0;
          0, d2(2)*sin(q2(2))];


    Ar = [cos(q1(1) + q1(2)), sin(q1(1) + q1(2));
          cos(q2(1) + q2(2)), sin(q2(1) + q2(2))];
    % forward model
    J = -pinv(Ar) * B;
    t0r = J * qda;
    % t0r =[ -(d1(2)*qd11*sin(q2(1) + q2(2))*sin(q1(2)) - ...
    %                 d2(2)*qd21*sin(q1(1) + q1(2))*sin(q2(2)))/sin(q1(1) + q1(2) - q2(1) - q2(2));
    %         (d1(2)*qd11*cos(q2(1) + q2(2))*sin(q1(2)) - ...
    %                 d2(2)*qd21*cos(q1(1) + q1(2))*sin(q2(2)))/sin(q1(1) + q1(2) - q2(1) - q2(2))];

    Jinv = -pinv(B) * Ar;
%     qda = Jinv * t0r;
    % qda = [(xd*cos(q1(1) + q1(2)) + yd*sin(q1(1) + q1(2)))/(d1(2)*sin(q1(2)));
    %        (xd*cos(q2(1) + q2(2)) + yd*sin(q2(1) + q2(2)))/(d2(2)*sin(q2(2)))];

    % passive velocities calculation

    ay = cos(Phi)^2 / (x - d2(2)*cos(q2(1)) - d2(1));
    ax = - ((y-d2(2)*sin(q2(1)))*cos(Phi)^2) ...
           / (x - d2(2)*cos(q2(1)) - d2(1))^2;
    aq = -(d2(2) * ((x-d2(1))*cos(q2(1)) ...
          +y*sin(q2(1))-d2(2))*cos(Phi)^2) ...
          / (x - d2(2)*cos(q2(1)) - d2(1))^2;

    Psit = [1                     0
            0                     1
            0                     0
            0                     0
            0                     0
            (ax+aq*Jinv(2,1)) (ay+aq*Jinv(2,2))];

    Jt = [-sin(q1(1) + q1(2)),cos(q1(1) + q1(2));
            (ax + aq*Jinv(2,1)), (ay + aq*Jinv(2,2));
            -sin(q2(1) + q2(2)),cos(q2(1) + q2(2))];


    Jta = [ d1(3) + d1(2)*cos(q1(2)), 0;
            1,                0;
            0,      d2(3) + d2(2)*cos(q2(2))];

    Jtd = [ d1(3), 0,   0;
            1,   1,   0;
            0,   0, d2(3)];

    qdp = Jtd\(Jt * t0r - Jta * qda);
    qd = [qda(1);qdp(1);qdp(2);qda(2);qdp(3)];

== matlab function five_bar_model_v_1/five-bar-robot2/forward kinematics ==
  data: qa input; p output; assembly input; q output
function [p,q] = fkine5(qa, assembly)
% This function implement the forward kinematic model of a five bar robot
% @parm qa: active joint positions vector 2x1
% @parm assembly: assembly mode selecction 1 for + -1 for -
% @return p: p end-effector coordinate vector 2X1
% @return q: joint positon vector 5X1
    l = 0.205;
    d1 = [-0.125, l, l];
    d2 = [0.125, l, l];
    q11 = qa(1);
    q21 = qa(2);

    A12 = [d1(2)*cos(q11)+d1(1); d1(2)*sin(q11)];
    A22 = [d2(2)*cos(q21)+d2(1); d2(2)*sin(q21)];

    if sqrt((A12-A22)' * (A12-A22)) <= 2*l
        a1 = - 2*d1(1) - 2*d1(2)*cos(q11);
        a2 = - 2*d2(1) - 2*d2(2)*cos(q21);
        b1 = - 2*sin(q11)*d1(2);
        b2 = - 2*sin(q21)*d2(2);
        c1 = d1(1)^2 + 2*cos(q11)*d1(1)*d1(2) + d1(2)^2 - d1(3)^2;
        c2 = d2(1)^2 + 2*cos(q21)*d2(1)*d2(2) + d2(2)^2 - d2(3)^2;

        if b1 ~= b2
            a = a2 - a1;
            b = b2 - b1;
            c = c2 - c1;
            e1 = - a / b;
            e2 = - c / b;
            f1 = 1 + e1^2;
            f2 = 2 * e1 * e2 + a1 + b1 * e1;
            f3 = e2^2 + b1 * e2 + c1;

            x = (-f2 - sqrt(f2^2 - 4 * f1 * f3)) / (2 * f1);
            y = e1 * x + e2;

            A13=[x-A12(1);y-A12(2)];
            A23=[x-A22(1);y-A22(2)];
            if  A13(1)*A23(2)-A23(1)*A13(2) <= 0 && assembly == 1
                x = (-f2 + sqrt(f2^2 - 4 * f1 * f3)) / (2 * f1);
                y = e1 * x + e2;
            elseif  A13(1)*A23(2)-A23(1)*A13(2) >= 0 && assembly == -1
                x = (-f2 + sqrt(f2^2 - 4 * f1 * f3)) / (2 * f1);
                y = e1 * x + e2;
            end
        else
            x = - (c2 - c1) / (a2 - a1);
            y = (-b1 + (b1^2 - 4 * (x^2 + a1 * x + c1))^(1/2)) / 2;

            A13=[x-A12(1);y-A12(2)];
            A23=[x-A22(1);y-A22(2)];
            if  A13(1)*A23(2)-A23(1)*A13(2) <= 0 && assembly == 1
                y = (-b1 - (b1^2 - 4 * (x^2 + a1 * x + c1))^(1/2)) / 2;
            elseif  A13(1)*A23(2)-A23(1)*A13(2) >= 0 && assembly == -1
                y = (-b1 - (b1^2 - 4 * (x^2 + a1 * x + c1))^(1/2)) / 2;
            end
        end

        % for q12 and q22 from a12/a11 and a22/a21
        q12 = atan2(y-d1(2)*sin(q11), x-d1(1)-d1(2)*cos(q11)) - q11;
        q22 = atan2(y-d2(2)*sin(q21), x-d2(1)-d2(2)*cos(q21)) - q21;
        q13 = q21 + q22 - q11 - q12;
        p = [x;y];
        q = [q11; q12; q13; q21; q22];
        
        % I will work in the first assembly.
        % Note: A way of implement the change of assembly is using the equations
        % (3) and (4) of the paper Minimum-time trajectory planning and control
        % of a pick-and-place five-bar parallel robot. Obtaining the
        % previous assembly, then the current and finally comparing
        % eache other.
%         sum(angdiff(q, q_prev).^2)
%         if sum(angdiff(q, q_prev).^2) > 0.1 
%             disp('Atention!!');
%             assembly2 = -assembly;
%             q11 = qa(1);
%             q21 = qa(2);
%             a1 = - 2*d1(1) - 2*d1(2)*cos(q11);
%             a2 = - 2*d2(1) - 2*d2(2)*cos(q21);
%             b1 = - 2*sin(q11)*d1(2);
%             b2 = - 2*sin(q21)*d2(2);
%             c1 = d1(1)^2 + 2*cos(q11)*d1(1)*d1(2) + d1(2)^2 - d1(3)^2;
%             c2 = d2(1)^2 + 2*cos(q21)*d2(1)*d2(2) + d2(2)^2 - d2(3)^2;
% 
%             if b1 ~= b2
%                 a = a2 - a1;
%                 b = b2 - b1;
%                 c = c2 - c1;
%                 e1 = - a / b;
%                 e2 = - c / b;
%                 f1 = 1 + e1^2;
%                 f2 = 2 * e1 * e2 + a1 + b1 * e1;
%                 f3 = e2^2 + b1 * e2 + c1;
% 
%                 x = (-f2 - sqrt(f2^2 - 4 * f1 * f3)) / (2 * f1);
%                 y = e1 * x + e2;
% 
%                 A13=[x-A12(1);y-A12(2)];
%                 A23=[x-A22(1);y-A22(2)];
%                 if  A13(1)*A23(2)-A23(1)*A13(2) <= 0 && assembly2 == 1
%                     x = (-f2 + sqrt(f2^2 - 4 * f1 * f3)) / (2 * f1);
%                     y = e1 * x + e2;
%                 elseif  A13(1)*A23(2)-A23(1)*A13(2) >= 0 && assembly2 == -1
%                     x = (-f2 + sqrt(f2^2 - 4 * f1 * f3)) / (2 * f1);
%                     y = e1 * x + e2;
%                 end
%             else
%                 x = - (c2 - c1) / (a2 - a1);
%                 y = (-b1 + (b1^2 - 4 * (x^2 + a1 * x + c1))^(1/2)) / 2;
% 
%                 A13=[x-A12(1);y-A12(2)];
%                 A23=[x-A22(1);y-A22(2)];
%                 if  A13(1)*A23(2)-A23(1)*A13(2) <= 0 && assembly == 1
%                     y = (-b1 - (b1^2 - 4 * (x^2 + a1 * x + c1))^(1/2)) / 2;
%                 elseif  A13(1)*A23(2)-A23(1)*A13(2) >= 0 && assembly == -1
%                     y = (-b1 - (b1^2 - 4 * (x^2 + a1 * x + c1))^(1/2)) / 2;
%                 end
%             end
% 
%             % for q12 and q22 from a12/a11 and a22/a21
%             q12 = atan2(y-d1(2)*sin(q11), x-d1(1)-d1(2)*cos(q11)) - q11;
%             q22 = atan2(y-d2(2)*sin(q21), x-d2(1)-d2(2)*cos(q21)) - q21;
%             q13 = q21 + q22 - q11 - q12;
%             p = [x;y];
%             q = [q11; q12; q13; q21; q22];
%         end
    else
        disp('ERROR: Euclidian distance > 2*l');
        p = [NaN; NaN];
        q = [NaN; NaN; NaN; NaN; NaN];
    end

== matlab function five_bar_model_v_1/five-bar-robot2/second order inverse kinematics ==
  data: qdda input; qdd output; t0r input; p input; q input; qd input; Ar input; J input; Jinv input; Jt input; Jta input; Jtd input; Psit input; qddp output; t0rd output; Psit1 output; Psit2 output; atp output; ad output
function [qdd,qddp,t0rd,Psit1,Psit2,atp,ad] = passive_acc5(qdda,t0r,p,q,qd,Ar,J,Jinv,Jt,Jta,Jtd,Psit)
% This function implement the second-order inverse kinematics model of a five bar robot
% @param t0rd: derivate twist end-effector vector 2X1
% @param t0r: twist end-effector vector 2X1
% @param p: end-effector coordinate vector 2X1
% @param q: joint positions vector 5x1
% @param qd: velocity joints vector 5x1
% @param Ar: matrix 2x2 for computation of the dynamic model of the PKM
% @param B: matrix 2x2 for computation of the dynamic model of the PKM
% @param Jinv: inverse kinematic Jacobian matrix of the PKM
% @param Jt: crucial for computation of the dynamic model of the PKM.
% @param Jta: crucial for computation of the dynamic model of the PKM.
% @param Jtd: crucial for computation of the dynamic model of the PKM.
% @return qdd: acceleration joint vector 5x1
% @return qdda: active acceleration joints vector 2X1
% @return qddu: underactuated acceleration joints vector 3X1
% @return Psit1: matrix 2x6
% @return Psit2: matrix 1x6
% @return atp: acceleration using for dynamics
% @return ad: acceleration using for dynamics

    l = 0.205;
    d1 = [-0.125, l, l];
    d2 = [0.125, l, l];
    q1 = q(1:3);
    q2 = q(4:5);
    qd1 = qd(1:3);
    qd2 = qd(4:5);
    Phi = sum(q1);
    Phid = sum(qd1);
    x = p(1);
    y = p(2);
    xd = t0r(1);
    yd = t0r(2);

    wr1 = [cos(q1(1)+q1(2)); sin(q1(1)+q1(2)); 0; 0; 0; 0];
    wr2 = [cos(q2(1)+q2(2)); sin(q2(1)+q2(2)); 0; 0; 0; 0];

    b01a_ = [-d1(2)*qd1(1)*cos(q1(1)) - d1(3)*cos(q1(1)+q1(2))*(qd1(1)+qd1(2));
             -d1(2)*qd1(1)*sin(q1(1)) - d1(3)*sin(q1(1)+q1(2))*(qd1(1)+qd1(2));
             zeros(4,1)];
    b01b_ = [-d1(3)*cos(q1(1)+q1(2));
             -d1(3)*sin(q1(1)+q1(2));
             zeros(4,1)];
    b0p1 = b01a_ * qd1(1) + b01b_ * qd1(2)*(qd1(1)+qd1(2));

    b02a_ = [-d2(2)*qd2(1)*cos(q2(1)) - d2(3)*cos(q2(1)+q2(2))*(qd2(1)+qd2(2));
             -d2(2)*qd2(1)*sin(q2(1)) - d2(3)*sin(q2(1)+q2(2))*(qd2(1)+qd2(2));
             zeros(4,1)];
    b02b_ = [-d2(3)*cos(q2(1)+q2(2));
             -d2(3)*sin(q2(1)+q2(2));
             zeros(4,1)];
    b0p2 = b02a_ * qd2(1) + b02b_ * qd2(2)*(qd2(1)+qd2(2));

    b0p = [(wr1'*b0p1); (wr2'*b0p2)];

%     aqq = pinv(B) * b0p;
    at = pinv(Ar) * b0p;
    t0rd = (J * qdda + at);
%     qdda = (Jinv * t0rd + aqq);

    % Aceleracion pasiva

    ayd = (Phid*sin(2*Phi))/(d2(1) - x + d2(2)*cos(q2(1))) - (cos(Phi)^2*(xd + d2(2)*qd2(1)*sin(q2(1))))/(d2(1) - x + d2(2)*cos(q2(1)))^2;

    axd = (Phid*sin(2*Phi)*(y - d2(2)*sin(q2(1))))/(d2(1) - x + d2(2)*cos(q2(1)))^2 ...
        - (cos(Phi)^2*(yd - d2(2)*qd2(1)*cos(q2(1))))/(d2(1) - x + d2(2)*cos(q2(1)))^2 ...
        - (2*cos(Phi)^2*(xd + d2(2)*qd2(1)*sin(q2(1)))*(y - d2(2)*sin(q2(1))))/(d2(1) - x + d2(2)*cos(q2(1)))^3;

    aqd = (2*d2(2)*cos(Phi)^2*(xd + d2(2)*qd2(1)*sin(q2(1)))*(d2(2) - sin(q2(1))*y + cos(q2(1))*(d2(1) - x)))...
        /(d2(1) - x + d2(2)*cos(q2(1)))^3 ...
        - (d2(2)*cos(Phi)^2*(xd*cos(q2(1)) + yd*sin(q2(1)) + qd2(1)*cos(q2(1))*y + qd2(1)*sin(q2(1))*(d2(1) - x)))...
        /(d2(1) - x + d2(2)*cos(q2(1)))^2 ...
        - (2*Phid*d2(2)*cos(Phi)*sin(Phi)*(d2(2) - sin(q2(1))*y + cos(q2(1))*(d2(1) - x)))...
        /(d2(1) - x + d2(2)*cos(q2(1)))^2;

    j21_invd = -(sin(q2(1) + q2(2))*(qd2(1) + qd2(2)))/(d2(2)*sin(q2(2))) ...
               -(qd2(2)*cos(q2(1) + q2(2))*cos(q2(2)))/(d2(2)*sin(q2(2))^2);

    j22_invd = -(qd2(2)*sin(q2(1) + q2(2))*cos(q2(2)))/(d2(2)*sin(q2(2))^2) ...
               +(cos(q2(1) + q2(2))*(qd2(1) + qd2(2)))/(d2(2)*sin(q2(2)));

    aq = -(d2(2) * ((x-d2(1))*cos(q2(1))+y*sin(q2(1))-d2(2))*cos(Phi)^2) / (x - d2(2)*cos(q2(1)) - d2(1))^2;

    psitd1 = axd + aqd*Jinv(2,1)+ aq*j21_invd;
    psitd2 = ayd + aqd*Jinv(2,2)+ aq*j22_invd;

    Psidt = [0 0; 0 0; 0 0; 0 0; 0 0; psitd1 psitd2];

    Psit1 = [-sin(q1(1)+q1(2)) cos(q1(1)+q1(2)) 0 0 0 0
             0                 0                0 0 0 1];
    Psit2 = [-sin(q2(1)+q2(2)) cos(q2(1)+q2(2)) 0 0 0 0];

    dc1 = Psit1 * (eye(6)* Psidt * t0r - b0p1); % Jti = I6x6 -> di = 06x1
    dc2 = Psit2 * (eye(6)* Psidt * t0r - b0p2);
    dc = [dc1; dc2];

    qddp =  Jtd\(Jt*t0rd - Jta*qdda + dc);

    qdd = [qdda(1);qddp(1);qddp(2);qdda(2);qddp(3)];

    at = pinv(Ar) * b0p;
    atp = Psit * at + Psidt * t0r;% using for dynamics
    ad = Jtd \ (dc + Jt*at); % For dynamics
